simulink model "Grid_2"  (R2016b)
settings: Solver=ode3  StartTime=0.0  StopTime=10.0  RelTol=1e-3
values from neighbouring files (symbols this model uses):
  Ts = 80e-6*2    (= 0.00016)    [initSimScript.m]
undefined symbols (not defined in the file or in its folder): Freq, Td
libraries: cables_lib x13, transformer_lib x7, modbus_lib x6, powerlib x5, dynamic_load_lib x4, Batt_lib x1, powerlib_meascontrol x1, PV_lib x1
settings Model: Creator=jlesage  LastModifiedBy=ch24070
settings DataIOCC: SaveFormat=StructureWithTime  SaveOutput=off  SaveTime=off
settings OptimizationCC: DefaultParameterBehavior=Inlined
settings HardwareCC: TargetBitPerPointer=64  TargetBitPerSizeT=64  TargetBitPerPtrDiffT=64  TargetLongLongMode=on  TargetIntDivRoundTo=Zero  TargetEndianess=LittleEndian  TargetWordSize=64  TargetHWDeviceType=MATLAB Host  ProdEqTarget=off
settings ModelReferenceCC: ModelReferenceNumInstancesAllowed=Single

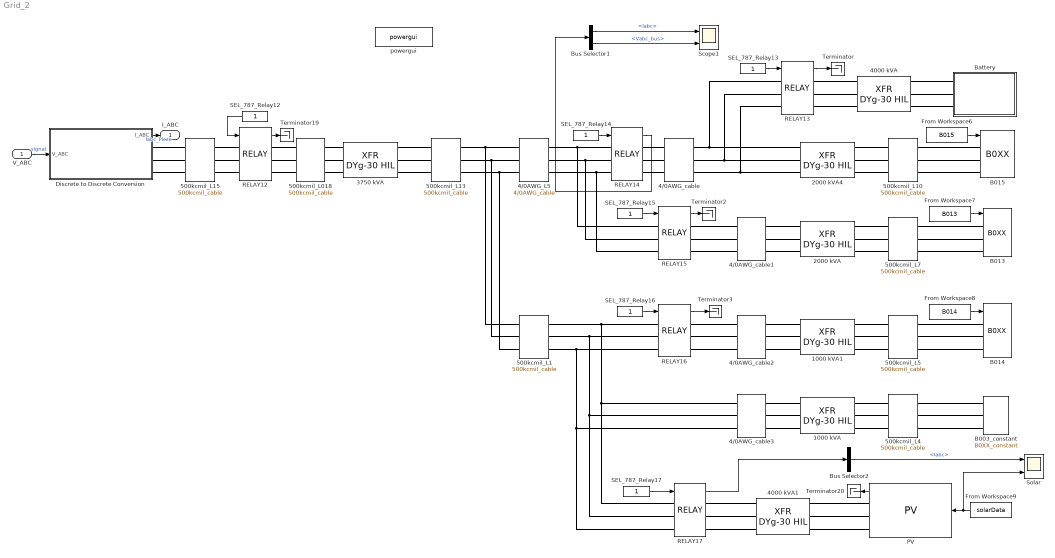
== system Grid_2 ==
  V_ABC : Inport  OutDataTypeStr=double  PortDimensions=3  SampleTime=Ts
  1000 kVA : transformer_lib/XFR DYg-30 HIL  Rating=1000  Vp=4160  Vs=460  Z=5.18  XR=2.5
  1000 kVA1 : transformer_lib/XFR DYg-30 HIL  Rating=1000  Vp=4160  Vs=216  Z=5.18  XR=2.5
  2000 kVA : transformer_lib/XFR DYg-30 HIL  Rating=2000  Vp=4160  Vs=216  Z=5.18  XR=2.5
  2000 kVA4 : transformer_lib/XFR DYg-30 HIL  Rating=2000  Vp=4160  Vs=216  Z=5.18  XR=2.5
  3750 kVA : transformer_lib/XFR DYg-30 HIL  Rating=3750  Vp=13800  Vs=4160  Z=4.75  XR=11.4
  4/0AWG_L5 : cables_lib/4//0AWG_cable  length=20  par_sets=1
  4/0AWG_cable{,1..3} (4 alike) : cables_lib/4//0AWG_cable  length=51  par_sets=1
  4000 kVA : transformer_lib/XFR DYg-30 HIL  Rating=4000  Vp=2047  Vs=4160  Z=6.37  XR=3.5
  4000 kVA1 : transformer_lib/XFR DYg-30 HIL  Rating=4000  Vp=2047  Vs=4160  Z=6.37  XR=3.5
  500kcmil_L018 : cables_lib/500kcmil_cable  length=1851  par_sets=1
  500kcmil_L1 : cables_lib/500kcmil_cable  length=50  par_sets=1
  500kcmil_L{4..5,7,10} (4 alike) : cables_lib/500kcmil_cable  length=25  par_sets=1
  500kcmil_L13 : cables_lib/500kcmil_cable  length=51  par_sets=1
  500kcmil_L15 : cables_lib/500kcmil_cable  length=50  par_sets=1
  B003_constant : dynamic_load_lib/B0XX_constant  v=460  kVA=60  pf=0.9
  B013 : dynamic_load_lib/B0XX  V=208  P_Scale=2  Q_Scale=2
  B014 : dynamic_load_lib/B0XX  V=208  P_Scale=1  Q_Scale=1
  B015 : dynamic_load_lib/B0XX  V=208  P_Scale=2  Q_Scale=2
  Battery : Subsystem
  Bus Selector1 : BusSelector  OutputSignals=Iabc,Vabc_bus
  Bus Selector2 : BusSelector  OutputSignals=Iabc
  Discrete to Discrete Conversion : Subsystem
  From Workspace6 : FromWorkspace  VariableName=B015  SampleTime=Ts  OutputAfterFinalValue=Holding final value
  From Workspace7 : FromWorkspace  VariableName=B013  SampleTime=Ts  OutputAfterFinalValue=Holding final value
  From Workspace8 : FromWorkspace  VariableName=B014  SampleTime=Ts  OutputAfterFinalValue=Holding final value
  From Workspace9 : FromWorkspace  VariableName=solarData  SampleTime=Ts  OutputAfterFinalValue=Holding final value
  PV : PV_lib/PV  max_power=4e6  VacRMS=1200  VacRMS_limit_pu=[1.15 0.85]
  RELAY12 : modbus_lib/RELAY  Ts=Ts
      link override Three-Phase V-I Measurement/Model/VI/Ia: GotoTag=LibraryTag_Ia
      link override Three-Phase V-I Measurement/Model/VI/Ib: GotoTag=LibraryTag_Ib
      link override Three-Phase V-I Measurement/Model/VI/Ic: GotoTag=LibraryTag_Ic
      link override Three-Phase V-I Measurement/Model/VI/Va: GotoTag=LibraryTag_Va
      link override Three-Phase V-I Measurement/Model/VI/Vb: GotoTag=LibraryTag_Vb
      link override Three-Phase V-I Measurement/Model/VI/Vc: GotoTag=LibraryTag_Vc
      link override Three-Phase V-I Measurement1/Model/VI/Ia: GotoTag=LibraryTag_Ia
      link override Three-Phase V-I Measurement1/Model/VI/Ib: GotoTag=LibraryTag_Ib
      link override Three-Phase V-I Measurement1/Model/VI/Ic: GotoTag=LibraryTag_Ic
      link override Three-Phase V-I Measurement1/Model/VI/Va: GotoTag=LibraryTag_Va
      link override Three-Phase V-I Measurement1/Model/VI/Vb: GotoTag=LibraryTag_Vb
      link override Three-Phase V-I Measurement1/Model/VI/Vc: GotoTag=LibraryTag_Vc
  RELAY13 : modbus_lib/RELAY  Ts=Ts
  RELAY14 : modbus_lib/RELAY  Ts=Ts
      link override Three-Phase V-I Measurement/Model/VI/Ia: GotoTag=LibraryTag_Ia
      link override Three-Phase V-I Measurement/Model/VI/Ib: GotoTag=LibraryTag_Ib
      link override Three-Phase V-I Measurement/Model/VI/Ic: GotoTag=LibraryTag_Ic
      link override Three-Phase V-I Measurement/Model/VI/Va: GotoTag=LibraryTag_Va
      link override Three-Phase V-I Measurement/Model/VI/Vb: GotoTag=LibraryTag_Vb
      link override Three-Phase V-I Measurement/Model/VI/Vc: GotoTag=LibraryTag_Vc
      link override Three-Phase V-I Measurement1/Model/VI/Ia: GotoTag=LibraryTag_Ia
      link override Three-Phase V-I Measurement1/Model/VI/Ib: GotoTag=LibraryTag_Ib
      link override Three-Phase V-I Measurement1/Model/VI/Ic: GotoTag=LibraryTag_Ic
      link override Three-Phase V-I Measurement1/Model/VI/Va: GotoTag=LibraryTag_Va
      link override Three-Phase V-I Measurement1/Model/VI/Vb: GotoTag=LibraryTag_Vb
      link override Three-Phase V-I Measurement1/Model/VI/Vc: GotoTag=LibraryTag_Vc
  RELAY15 : modbus_lib/RELAY  Ts=Ts
      link override Three-Phase V-I Measurement/Model/VI/Ia: GotoTag=LibraryTag_Ia
      link override Three-Phase V-I Measurement/Model/VI/Ib: GotoTag=LibraryTag_Ib
      link override Three-Phase V-I Measurement/Model/VI/Ic: GotoTag=LibraryTag_Ic
      link override Three-Phase V-I Measurement/Model/VI/Va: GotoTag=LibraryTag_Va
      link override Three-Phase V-I Measurement/Model/VI/Vb: GotoTag=LibraryTag_Vb
      link override Three-Phase V-I Measurement/Model/VI/Vc: GotoTag=LibraryTag_Vc
      link override Three-Phase V-I Measurement1/Model/VI/Ia: GotoTag=LibraryTag_Ia
      link override Three-Phase V-I Measurement1/Model/VI/Ib: GotoTag=LibraryTag_Ib
      link override Three-Phase V-I Measurement1/Model/VI/Ic: GotoTag=LibraryTag_Ic
      link override Three-Phase V-I Measurement1/Model/VI/Va: GotoTag=LibraryTag_Va
      link override Three-Phase V-I Measurement1/Model/VI/Vb: GotoTag=LibraryTag_Vb
      link override Three-Phase V-I Measurement1/Model/VI/Vc: GotoTag=LibraryTag_Vc
  RELAY16 : modbus_lib/RELAY  Ts=Ts
      link override Three-Phase V-I Measurement/Model/VI/Ia: GotoTag=LibraryTag_Ia
      link override Three-Phase V-I Measurement/Model/VI/Ib: GotoTag=LibraryTag_Ib
      link override Three-Phase V-I Measurement/Model/VI/Ic: GotoTag=LibraryTag_Ic
      link override Three-Phase V-I Measurement/Model/VI/Va: GotoTag=LibraryTag_Va
      link override Three-Phase V-I Measurement/Model/VI/Vb: GotoTag=LibraryTag_Vb
      link override Three-Phase V-I Measurement/Model/VI/Vc: GotoTag=LibraryTag_Vc
      link override Three-Phase V-I Measurement1/Model/VI/Ia: GotoTag=LibraryTag_Ia
      link override Three-Phase V-I Measurement1/Model/VI/Ib: GotoTag=LibraryTag_Ib
      link override Three-Phase V-I Measurement1/Model/VI/Ic: GotoTag=LibraryTag_Ic
      link override Three-Phase V-I Measurement1/Model/VI/Va: GotoTag=LibraryTag_Va
      link override Three-Phase V-I Measurement1/Model/VI/Vb: GotoTag=LibraryTag_Vb
      link override Three-Phase V-I Measurement1/Model/VI/Vc: GotoTag=LibraryTag_Vc
  RELAY17 : modbus_lib/RELAY  Ts=Ts
      link override Three-Phase V-I Measurement/Model/VI/Ia: GotoTag=LibraryTag_Ia
      link override Three-Phase V-I Measurement/Model/VI/Ib: GotoTag=LibraryTag_Ib
      link override Three-Phase V-I Measurement/Model/VI/Ic: GotoTag=LibraryTag_Ic
      link override Three-Phase V-I Measurement/Model/VI/Va: GotoTag=LibraryTag_Va
      link override Three-Phase V-I Measurement/Model/VI/Vb: GotoTag=LibraryTag_Vb
      link override Three-Phase V-I Measurement/Model/VI/Vc: GotoTag=LibraryTag_Vc
      link override Three-Phase V-I Measurement1/Model/VI/Ia: GotoTag=LibraryTag_Ia
      link override Three-Phase V-I Measurement1/Model/VI/Ib: GotoTag=LibraryTag_Ib
      link override Three-Phase V-I Measurement1/Model/VI/Ic: GotoTag=LibraryTag_Ic
      link override Three-Phase V-I Measurement1/Model/VI/Va: GotoTag=LibraryTag_Va
      link override Three-Phase V-I Measurement1/Model/VI/Vb: GotoTag=LibraryTag_Vb
      link override Three-Phase V-I Measurement1/Model/VI/Vc: GotoTag=LibraryTag_Vc
  SEL_787_Relay{12..17} (6 alike) : Constant
  Scope1 : Scope  NumInputPorts=2
  Solar : Scope  NumInputPorts=2
  Terminator{,2..3,19..20} (5 alike) : Terminator
  powergui : powerlib/powergui  Priority=2  SimulationMode=Discrete  SolverType=Tustin/Backward Euler (TBE)  SampleTime=Ts  frequency=60  SPID=off  DisableSnubberDevices=off  DisableRonSwitches=off  DisableVfSwitches=off  SwTol=0  DisplayEquations=off  Interpol=off  ExternalGateDelay=off  methode=off  Ts=0  FunctionMessages=off  echomessages=off  HookPort=off  EnableUseOfTLC=on  x0status=blocks  frequencyindice=0  Pbase=100e6  ErrMax=1e-4  Iterations=50  UnitsV=kV  UnitsW=MW  buscounter=0  RestoreLinks=warning  ResistiveCurrentMeasurement=off  Frange=logspace(0,3,50)  Ylog=off  Xlog=off  ShowGrid=off  save=off  variable=ZData  structure=0  ZoomFFT=on  StartTime=0.0  cycles=2  DisplayStyle=off  fundamental=60  FreqAxis=off  MaxFrequency=1000  frequencyindicesteady=1  RmsSteady=1  display=off
  I_ABC : Outport  OutDataTypeStr=double  PortDimensions=3  SampleTime=Ts
  wires:
  From Workspace9/1 -> PV/1, Solar/2
  From Workspace7/1 -> B013/1
  SEL_787_Relay15/1 -> RELAY15/1
  SEL_787_Relay14/1 -> RELAY14/1
  RELAY15/1 -> Terminator2/1
  SEL_787_Relay13/1 -> RELAY13/1
  From Workspace6/1 -> B015/1
  RELAY13/1 -> Terminator/1
  From Workspace8/1 -> B014/1
  RELAY16/1 -> Terminator3/1
  SEL_787_Relay16/1 -> RELAY16/1
  RELAY17/1 -> Bus Selector2/1
  SEL_787_Relay17/1 -> RELAY17/1
  RELAY12/1 -> Terminator19/1
  SEL_787_Relay12/1 -> RELAY12/1
  PV/1 -> Terminator20/1
  RELAY14/1 -> Bus Selector1/1
  Bus Selector1/1 -> Scope1/1  "<Iabc>"
  Bus Selector1/2 -> Scope1/2  "<Vabc_bus>"
  Bus Selector2/1 -> Solar/1  "<Iabc>"
  Discrete to Discrete Conversion/1(I_ABC) -> I_ABC/1  "Iabc_Piece"
  V_ABC/1 -> Discrete to Discrete Conversion/1(V_ABC)  "signal"
  connections:
  RELAY14/LConn3 -- RELAY15/LConn3 -- 4/0AWG_L5/RConn3
  RELAY14/LConn2 -- RELAY15/LConn2 -- 4/0AWG_L5/RConn2
  RELAY14/LConn1 -- RELAY15/LConn1 -- 4/0AWG_L5/RConn1
  4/0AWG_cable3/LConn3 -- 500kcmil_L1/RConn3 -- RELAY16/LConn3 -- RELAY17/LConn3
  4/0AWG_cable3/LConn1 -- RELAY16/LConn1 -- 500kcmil_L1/RConn1 -- RELAY17/LConn1
  4/0AWG_cable/RConn3 -- RELAY13/LConn3 -- 2000 kVA4/LConn3
  4/0AWG_cable/RConn2 -- RELAY13/LConn2 -- 2000 kVA4/LConn2
  4/0AWG_cable/RConn1 -- RELAY13/LConn1 -- 2000 kVA4/LConn1
  4/0AWG_cable3/LConn2 -- 500kcmil_L1/RConn2 -- RELAY16/LConn2 -- RELAY17/LConn2
  500kcmil_L13/RConn3 -- 4/0AWG_L5/LConn3 -- 500kcmil_L1/LConn3
  500kcmil_L13/RConn2 -- 4/0AWG_L5/LConn2 -- 500kcmil_L1/LConn2
  500kcmil_L13/RConn1 -- 4/0AWG_L5/LConn1 -- 500kcmil_L1/LConn1
  RELAY14/RConn3 -- 4/0AWG_cable/LConn3
  RELAY14/RConn1 -- 4/0AWG_cable/LConn1
  4000 kVA1/LConn3 -- PV/RConn3
  4000 kVA1/LConn2 -- PV/RConn2
  4000 kVA1/LConn1 -- PV/RConn1
  RELAY14/RConn2 -- 4/0AWG_cable/LConn2
  500kcmil_L10/RConn1 -- B015/LConn1
  500kcmil_L7/RConn2 -- B013/LConn2
  500kcmil_L10/RConn2 -- B015/LConn2
  500kcmil_L7/RConn1 -- B013/LConn1
  500kcmil_L10/RConn3 -- B015/LConn3
  RELAY15/RConn2 -- 4/0AWG_cable1/LConn2
  500kcmil_L4/RConn1 -- B003_constant/LConn1
  2000 kVA4/RConn3 -- 500kcmil_L10/LConn3
  4/0AWG_cable1/RConn1 -- 2000 kVA/LConn1
  500kcmil_L4/RConn3 -- B003_constant/LConn3
  4/0AWG_cable1/RConn2 -- 2000 kVA/LConn2
  RELAY16/RConn3 -- 4/0AWG_cable2/LConn3
  500kcmil_L5/LConn2 -- 1000 kVA1/RConn2
  RELAY16/RConn1 -- 4/0AWG_cable2/LConn1
  500kcmil_L4/LConn3 -- 1000 kVA/RConn3
  500kcmil_L4/RConn2 -- B003_constant/LConn2
  1000 kVA1/LConn3 -- 4/0AWG_cable2/RConn3
  4/0AWG_cable1/LConn3 -- RELAY15/RConn3
  4/0AWG_cable2/LConn2 -- RELAY16/RConn2
  500kcmil_L5/LConn1 -- 1000 kVA1/RConn1
  500kcmil_L7/LConn2 -- 2000 kVA/RConn2
  500kcmil_L5/LConn3 -- 1000 kVA1/RConn3
  1000 kVA1/LConn1 -- 4/0AWG_cable2/RConn1
  500kcmil_L7/LConn3 -- 2000 kVA/RConn3
  4/0AWG_cable1/LConn1 -- RELAY15/RConn1
  4/0AWG_cable1/RConn3 -- 2000 kVA/LConn3
  500kcmil_L7/LConn1 -- 2000 kVA/RConn1
  1000 kVA1/LConn2 -- 4/0AWG_cable2/RConn2
  2000 kVA4/RConn2 -- 500kcmil_L10/LConn2
  500kcmil_L4/LConn2 -- 1000 kVA/RConn2
  2000 kVA4/RConn1 -- 500kcmil_L10/LConn1
  500kcmil_L5/RConn1 -- B014/LConn1
  500kcmil_L5/RConn2 -- B014/LConn2
  500kcmil_L7/RConn3 -- B013/LConn3
  RELAY13/RConn3 -- 4000 kVA/RConn3
  500kcmil_L4/LConn1 -- 1000 kVA/RConn1
  1000 kVA/LConn2 -- 4/0AWG_cable3/RConn2
  RELAY17/RConn2 -- 4000 kVA1/RConn2
  RELAY17/RConn1 -- 4000 kVA1/RConn1
  1000 kVA/LConn3 -- 4/0AWG_cable3/RConn3
  RELAY17/RConn3 -- 4000 kVA1/RConn3
  1000 kVA/LConn1 -- 4/0AWG_cable3/RConn1
  500kcmil_L5/RConn3 -- B014/LConn3
  RELAY13/RConn2 -- 4000 kVA/RConn2
  RELAY13/RConn1 -- 4000 kVA/RConn1
  RELAY12/RConn3 -- 500kcmil_L018/LConn3
  500kcmil_L15/RConn3 -- RELAY12/LConn3
  500kcmil_L15/RConn1 -- RELAY12/LConn1
  RELAY12/RConn1 -- 500kcmil_L018/LConn1
  RELAY12/LConn2 -- 500kcmil_L15/RConn2
  RELAY12/RConn2 -- 500kcmil_L018/LConn2
  500kcmil_L13/LConn1 -- 3750 kVA/RConn1
  3750 kVA/RConn2 -- 500kcmil_L13/LConn2
  500kcmil_L018/RConn2 -- 3750 kVA/LConn2
  500kcmil_L018/RConn1 -- 3750 kVA/LConn1
  500kcmil_L13/LConn3 -- 3750 kVA/RConn3
  500kcmil_L018/RConn3 -- 3750 kVA/LConn3
  4000 kVA/LConn1 -- Battery/RConn1
  4000 kVA/LConn2 -- Battery/RConn2
  4000 kVA/LConn3 -- Battery/RConn3
  Discrete to Discrete Conversion/RConn1 -- 500kcmil_L15/LConn1
  Discrete to Discrete Conversion/RConn2 -- 500kcmil_L15/LConn2
  Discrete to Discrete Conversion/RConn3 -- 500kcmil_L15/LConn3

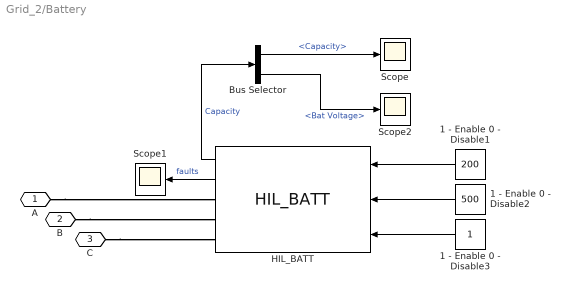
== system Grid_2/Battery ==
  1 - Enable 0 - Disable1 : Constant  Value=200
  1 - Enable 0 - Disable2 : Constant  Value=500
  1 - Enable 0 - Disable3 : Constant
  Bus Selector : BusSelector  OutputSignals=Capacity,Bat Voltage
  HIL_BATT : Batt_lib/HIL_BATT
  Scope : Scope
  Scope1 : Scope
  Scope2 : Scope
  A : PMIOPort  Port=1  Side=Right
  B : PMIOPort  Port=2  Side=Right
  C : PMIOPort  Port=3  Side=Right
  wires:
  Bus Selector/2 -> Scope2/1  "<Bat Voltage>"
  Bus Selector/1 -> Scope/1  "<Capacity>"
  HIL_BATT/2 -> Scope1/1  "faults"
  1 - Enable 0 - Disable3/1 -> HIL_BATT/3
  1 - Enable 0 - Disable1/1 -> HIL_BATT/1
  HIL_BATT/1 -> Bus Selector/1  "Capacity"
  1 - Enable 0 - Disable2/1 -> HIL_BATT/2
  connections:
  C/RConn1 -- HIL_BATT/RConn3
  B/RConn1 -- HIL_BATT/RConn2
  A/RConn1 -- HIL_BATT/RConn1

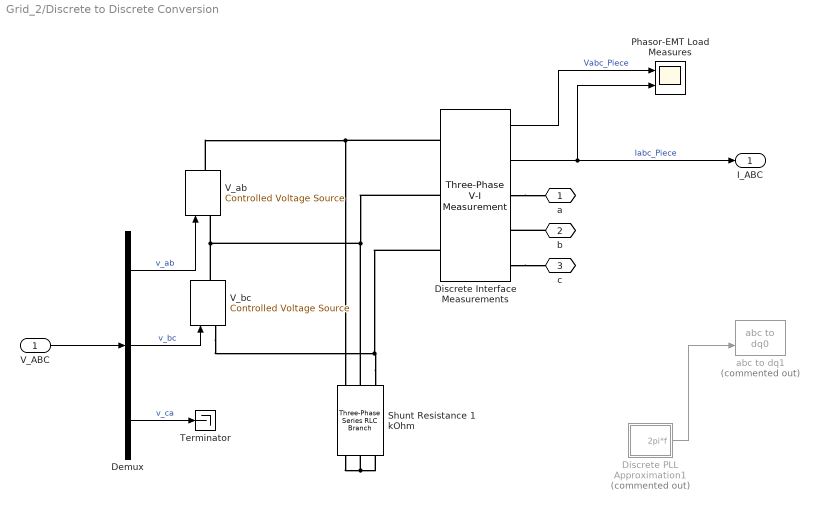
== system Grid_2/Discrete to Discrete Conversion ==
  V_ABC : Inport
  Demux : Demux  Outputs=3
  Discrete Interface Measurements : powerlib/Measurements/Three-Phase V-I Measurement  VoltageMeasurement=phase-to-phase  SetLabelV=off  LabelV=Vabc  Vpu=off  VpuLL=off  CurrentMeasurement=yes  SetLabelI=off  LabelI=Iabc  Ipu=off  Pbase=100e6  Vbase=500e3  OutputType=Complex  PhasorSimulation=off  PSBequivalent=0
  Discrete PLL Approximation1 : Subsystem  Commented=on
  Phasor-EMT Load Measures : Scope  NumInputPorts=2
  Shunt Resistance 1 kOhm : powerlib/Elements/Three-Phase Series RLC Branch  LConnTagsString=A|B|C  RConnTagsString=A|B|C  BranchType=R  Resistance=1e6  Inductance=1e-3  Capacitance=1e-6  Measurements=None
  Terminator : Terminator
  V_ab : powerlib/Electrical Sources/Controlled Voltage Source  Initialize=off  Source_Type=AC  Amplitude=0  Phase=0  Frequency=0  Measurements=None
  V_bc : powerlib/Electrical Sources/Controlled Voltage Source  Initialize=off  Source_Type=AC  Amplitude=0  Phase=0  Frequency=0  Measurements=None
  abc to dq1 : powerlib_meascontrol/Transformations/abc to dq0  Commented=on  Alignment=90 degrees behind phase A axis
  a : PMIOPort  Port=1  Side=Right
  b : PMIOPort  Port=2  Side=Right
  c : PMIOPort  Port=3  Side=Right
  I_ABC : Outport
  wires:
  Discrete PLL Approximation1/1(2pi*f) -> abc to dq1/2
  ? -> abc to dq1/1  "Iabc_Piece"
  Discrete Interface Measurements/2 -> Phasor-EMT Load Measures/2, I_ABC/1  "Iabc_Piece"
  Demux/3 -> Terminator/1  "v_ca"
  Discrete Interface Measurements/1 -> Phasor-EMT Load Measures/1  "Vabc_Piece"
  Demux/1 -> V_ab/1  "v_ab"
  Demux/2 -> V_bc/1  "v_bc"
  V_ABC/1 -> Demux/1
  connections:
  Shunt Resistance 1 kOhm/RConn2 -- Shunt Resistance 1 kOhm/RConn3 -- Shunt Resistance 1 kOhm/RConn1
  Shunt Resistance 1 kOhm/LConn3 -- Discrete Interface Measurements/LConn3 -- V_bc/LConn1
  Discrete Interface Measurements/LConn1 -- Shunt Resistance 1 kOhm/LConn1 -- V_ab/RConn1
  V_ab/LConn1 -- Shunt Resistance 1 kOhm/LConn2 -- Discrete Interface Measurements/LConn2 -- V_bc/RConn1
  Discrete Interface Measurements/RConn1 -- a/RConn1
  b/RConn1 -- Discrete Interface Measurements/RConn2
  Discrete Interface Measurements/RConn3 -- c/RConn1

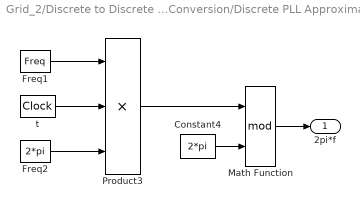
== system Grid_2/Discrete to Discrete Conversion/Discrete PLL Approximation1 ==
  Constant4 : Constant  Value=2*pi
  Freq1 : Constant  Value=Freq
  Freq2 : Constant  Value=2*pi
  Math Function : Math  Operator=mod  SaturateOnIntegerOverflow=on
  Product3 : Product  Inputs=***  SaturateOnIntegerOverflow=on  InputSameDT=on  OutDataTypeStr=Inherit: Same as first input
  t : DigitalClock  SampleTime=Td
  2pi*f : Outport
  wires:
  Math Function/1 -> 2pi*f/1
  Product3/1 -> Math Function/1
  Constant4/1 -> Math Function/2
  Freq1/1 -> Product3/1
  Freq2/1 -> Product3/3
  t/1 -> Product3/2
